simulink model "madde2_2"  (R2015b)
settings: Solver=VariableStepAuto  StartTime=0.0  StopTime=0.5  RelTol=1e-3
libraries: powerlib x10
settings Model: Creator=brownie  LastModifiedBy=brownie

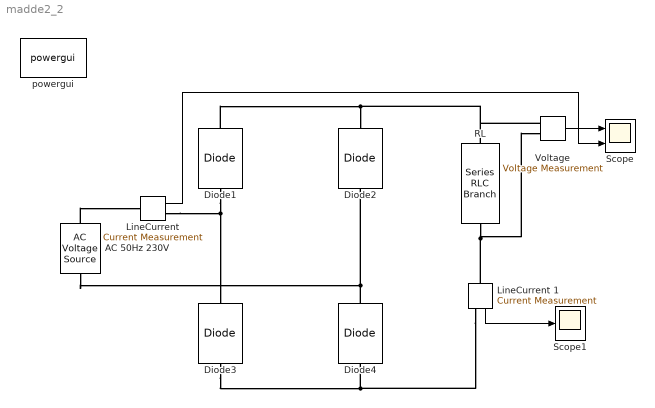
== system madde2_2 ==
  AC 50Hz 230V : powerlib/Electrical Sources/AC Voltage Source  Amplitude=325  Phase=0  Frequency=50  SampleTime=0  Measurements=None  BusType=swing  Pref=10e3  Qref=0  Qmin=-inf  Qmax=+inf
  Diode1 : powerlib/Power Electronics/Diode  Ron=0.00001  Lon=0  Vf=0  IC=0  UseSnubber=off  Rs=500  Cs=250e-9  Measurements=off
  Diode2 : powerlib/Power Electronics/Diode  Ron=0.0001  Lon=0  Vf=0  IC=0  UseSnubber=off  Rs=500  Cs=250e-9  Measurements=off
  Diode3 : powerlib/Power Electronics/Diode  Ron=0.0001  Lon=0  Vf=0  IC=0  UseSnubber=off  Rs=500  Cs=250e-9  Measurements=off
  Diode4 : powerlib/Power Electronics/Diode  Ron=0.0001  Lon=0  Vf=0  IC=0  UseSnubber=off  Rs=500  Cs=250e-9  Measurements=off
  "LineCurrent " : powerlib/Measurements/Current Measurement  PhasorSimulation=off  OutputType=Complex  PSBequivalent=0
  LineCurrent 1 : powerlib/Measurements/Current Measurement  PhasorSimulation=off  OutputType=Complex  PSBequivalent=0
  RL : powerlib/Elements/Series RLC Branch  LConnTagsString=__new0  RConnTagsString=__new0  BranchType=RL  Resistance=25  Inductance=1  SetiL0=off  InitialCurrent=0  Capacitance=5e-4  Setx0=off  InitialVoltage=0  Measurements=None
  Scope : Scope  NumInputPorts=2
  Scope1 : Scope
  Voltage : powerlib/Measurements/Voltage Measurement  PhasorSimulation=off  OutputType=Complex  PSBequivalent=0
  powergui : powerlib/powergui  Priority=1  SimulationMode=Discrete  SolverType=Backward Euler  SampleTime=1e-5  frequency=60  SPID=off  DisableSnubberDevices=off  DisableRonSwitches=off  DisableVfSwitches=off  SwTol=0  DisplayEquations=off  Interpol=off  ExternalGateDelay=off  methode=off  Ts=10  FunctionMessages=off  echomessages=off  HookPort=off  EnableUseOfTLC=off  x0status=blocks  frequencyindice=50  Pbase=100e6  ErrMax=1e-4  Iterations=50  UnitsV=kV  UnitsW=MW  buscounter=0  RestoreLinks=warning  ResistiveCurrentMeasurement=off  Frange=[0:2:500]  Ylog=off  Xlog=on  ShowGrid=off  save=off  variable=ZData  structure=ScopeData  ZoomFFT=off  StartTime=0.1  cycles=10  DisplayStyle=1  fundamental=50  FreqAxis=off  MaxFrequency=1000  frequencyindicesteady=1  RmsSteady=1  display=off
  wires:
  Voltage/1 -> Scope/1
  "LineCurrent "/1 -> Scope/2
  LineCurrent 1/1 -> Scope1/1
  connections:
  Diode4/RConn1 -- AC 50Hz 230V/LConn1 -- Diode2/LConn1
  Diode1/LConn1 -- Diode3/RConn1 -- "LineCurrent "/RConn1
  Diode3/LConn1 -- LineCurrent 1/RConn1 -- Diode4/LConn1
  Diode1/RConn1 -- RL/LConn1 -- Voltage/LConn1 -- Diode2/RConn1
  AC 50Hz 230V/RConn1 -- "LineCurrent "/LConn1
  RL/RConn1 -- Voltage/LConn2 -- LineCurrent 1/LConn1
